simulink model "model_linearization"  (R2014b)
settings: Solver=ode45  StartTime=0.0  StopTime=10.0  RelTol=1e-3
values from neighbouring files (symbols this model uses):
  states_IC = [      13.9 ... (first row only)    [startup.m]    (also in trim_model.m = [14.048)
undefined symbols (not defined in the file or in its folder): slparams
settings Model: Creator=thomas  LastModifiedBy=thomas

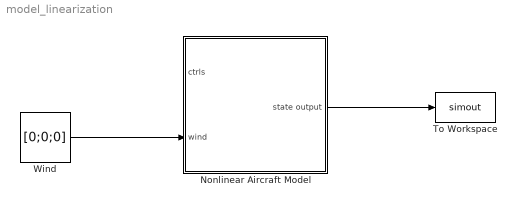
== system model_linearization ==
  Nonlinear Aircraft Model : Subsystem
  To Workspace : ToWorkspace  VariableName=simout  SampleTime=-1
  Wind : Constant  Value=[0;0;0]
  wires:
  Wind/1 -> Nonlinear Aircraft Model/2(wind)
  Nonlinear Aircraft Model/1(state output) -> To Workspace/1

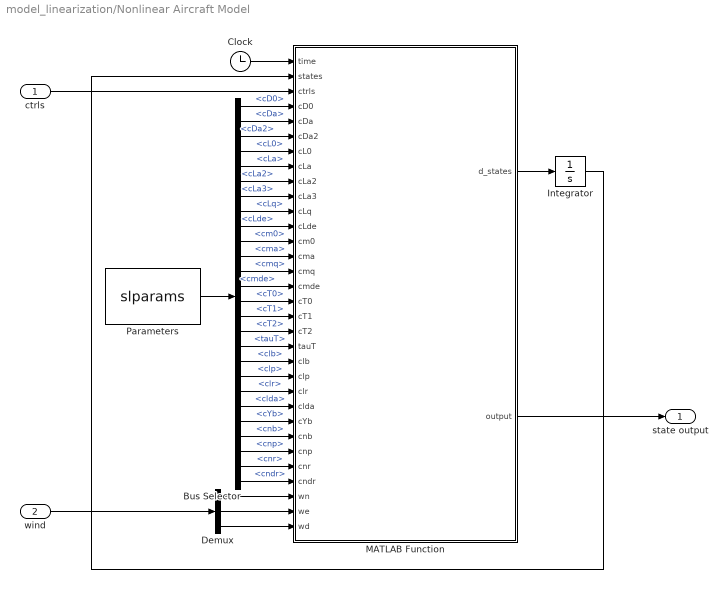
== system model_linearization/Nonlinear Aircraft Model ==
  ctrls : Inport
  wind : Inport  Port=2
  Bus Selector : BusSelector  OutputSignals=cD0,cDa,cDa2,cL0,cLa,cLa2,cLa3,cLq,cLde,cm0,cma,cmq,cmde,cT0,cT1,cT2,tauT,clb,clp,clr,clda,cYb,cnb,cnp,cnr,cndr
  Clock : Clock
  Demux : Demux  Outputs=3
  Integrator : Integrator  InitialCondition=states_IC
  MATLAB Function : MATLAB Function  TreatAsAtomicUnit=on
  Parameters : Constant  Value=slparams  OutDataTypeStr=Bus: slBus1
  state output : Outport
  wires:
  Bus Selector/3 -> MATLAB Function/6(cDa2)  "<cDa2>"
  Bus Selector/8 -> MATLAB Function/11(cLq)  "<cLq>"
  Bus Selector/5 -> MATLAB Function/8(cLa)  "<cLa>"
  Bus Selector/16 -> MATLAB Function/19(cT2)  "<cT2>"
  Bus Selector/13 -> MATLAB Function/16(cmde)  "<cmde>"
  Bus Selector/1 -> MATLAB Function/4(cD0)  "<cD0>"
  Bus Selector/17 -> MATLAB Function/20(tauT)  "<tauT>"
  Bus Selector/2 -> MATLAB Function/5(cDa)  "<cDa>"
  Bus Selector/11 -> MATLAB Function/14(cma)  "<cma>"
  Bus Selector/20 -> MATLAB Function/23(clr)  "<clr>"
  Bus Selector/21 -> MATLAB Function/24(clda)  "<clda>"
  Bus Selector/18 -> MATLAB Function/21(clb)  "<clb>"
  Bus Selector/15 -> MATLAB Function/18(cT1)  "<cT1>"
  Bus Selector/6 -> MATLAB Function/9(cLa2)  "<cLa2>"
  Bus Selector/4 -> MATLAB Function/7(cL0)  "<cL0>"
  Bus Selector/22 -> MATLAB Function/25(cYb)  "<cYb>"
  Bus Selector/26 -> MATLAB Function/29(cndr)  "<cndr>"
  Bus Selector/23 -> MATLAB Function/26(cnb)  "<cnb>"
  Bus Selector/10 -> MATLAB Function/13(cm0)  "<cm0>"
  Bus Selector/25 -> MATLAB Function/28(cnr)  "<cnr>"
  Bus Selector/9 -> MATLAB Function/12(cLde)  "<cLde>"
  Bus Selector/24 -> MATLAB Function/27(cnp)  "<cnp>"
  Bus Selector/19 -> MATLAB Function/22(clp)  "<clp>"
  Parameters/1 -> Bus Selector/1
  Bus Selector/7 -> MATLAB Function/10(cLa3)  "<cLa3>"
  Bus Selector/14 -> MATLAB Function/17(cT0)  "<cT0>"
  Bus Selector/12 -> MATLAB Function/15(cmq)  "<cmq>"
  MATLAB Function/1(d_states) -> Integrator/1
  ctrls/1 -> MATLAB Function/3(ctrls)
  Integrator/1 -> MATLAB Function/2(states)
  MATLAB Function/2(output) -> state output/1
  Clock/1 -> MATLAB Function/1(time)
  wind/1 -> Demux/1
  Demux/1 -> MATLAB Function/30(wn)
  Demux/2 -> MATLAB Function/31(we)
  Demux/3 -> MATLAB Function/32(wd)

== matlab function model_linearization/Nonlinear Aircraft Model/MATLAB Function ==
  data: time input; d_states output; states input; ctrls input; cD0 input; cDa input; cDa2 input; cL0 input; cLa input; cLa2 input; cLa3 input; cLq input; cLde input; cm0 input; cma input; cmq input; cmde input; cT0 input; cT1 input; cT2 input; tauT input; clb input; clp input; clr input; clda input; cYb input; cnb input; cnp input; cnr input; cndr input; wn input; we input; wd input; output output
function [d_states, output]  = NonlinearModel(time, states, ctrls,...
    cD0, cDa, cDa2, ...
    cL0, cLa, cLa2, cLa3, cLq, cLde, ...
    cm0, cma, cmq, cmde, ...
    cT0, cT1, cT2, tauT, ...
    clb, clp, clr, clda, ...
    cYb, ...
    cnb, cnp, cnr, cndr, ...
    wn, we, wd)

%#codegen
%--------------------------------------------------------------------------
% TECHPOD NONLINEAR 6DoF AIRCRAFT MODEL
%
% last update 07.06.15, Thomas Stastny

%--------------------------------------------------------------------------

% states
u       = states(1);    % x-body velocity
v       = states(2);    % y-body velocity
w       = states(3);    % z-body velocity

p       = states(4);    % roll rate
q       = states(5);    % pitch rate
r       = states(6);    % yaw rate

phi 	= states(7);    % roll angle
theta   = states(8);    % pitch angle
psi     = states(9);    % flight path angle

n       = states(10);   % inertial north position
e       = states(11);   % inertial east position
d       = states(12);   % inertial down position

uT      = states(13);

% controls
uTcmd      = ctrls(1);     % throttle
uE      = ctrls(2);     % elevator deflection
uA      = ctrls(3);     % aileron deflection (uniform)
uR      = ctrls(4);     % rudder deflection

if uTcmd>1, uTcmd=1; end;
if uTcmd<0, uTcmd=0; end;
if uE>20*pi/180, uE=20*pi/180; end;
if uE<-20*pi/180, uE=-20*pi/180; end;
if uA>20*pi/180, uA=20*pi/180; end;
if uA<-20*pi/180, uA=-20*pi/180; end;
if uR>20*pi/180, uR=20*pi/180; end;
if uR<-20*pi/180, uR=-20*pi/180; end;

% MODEL CONSTRUCTION ------------------------------------------------------

% intermediate states
V       = sqrt(u^2+v^2+w^2);
beta    = asin(v/V);
alpha   = atan(w/u);

% MODEL CONSTRUCTION ------------------------------------------------------

% geometry
S_wing          = 0.47;     % wing surface              [m^2]
b_wing          = 2.59;     % wingspan                  [m]
c_chord         = 0.180;    % mean chord length         [m]
i_thrust        = 0*pi/180;	% thrust incidence angle    [rad] -->NOTE: i is defined from body x in positive pitch (up)

% mass / inertia
mass    = 2.65;         % total mass of airplane    [kg]
Ixx     = 0.1512*1.1;	% inertias                  [kg m^2]
Iyy     = 0.2785*1.4;	% inertias                  [kg m^2]
Izz     = 0.3745*1.4;	% inertias                  [kg m^2]
Ixz     = 0.0755;       % inertias                  [kg m^2]

% environment
g       = 9.81;     % gravitational acceleration    [m/s^2]
rho_air = 1.18;     % air density

% wind to body transform
ca = cos(alpha);
sa = sin(alpha);
H_W2B = [ca,	0,	-sa;
         0,     1,	0;
         sa,    0,	ca];

% non-dimensionalization
p_hat	= p*b_wing /(2*V);
q_hat	= q*c_chord /(2*V);
r_hat	= r*b_wing /(2*V);
q_bar_S = 1/2*rho_air*V^2*S_wing;

% stability axis aerodynamic force coefficients
cD      = cD0 + cDa*alpha + cDa2*alpha^2;
cY_s    = cYb*beta;
cL      = cL0 + cLa*alpha + cLa2*alpha^2 + cLa3*alpha^3 + cLq*q_hat + cLde*uE;

% body frame aerodynamic forces
cXYZ    = H_W2B*[-cD; cY_s; -cL];
X       = q_bar_S * cXYZ(1);
Y       = q_bar_S * cXYZ(2);
Z       = q_bar_S * cXYZ(3);

% stability axis aerodynamic moment coefficients
cl_s    = clb*beta + clp*p_hat + clr*r_hat + clda*uA;
cm_s    = cm0 + cma*alpha + cmq*q_hat + cmde*uE;
cn_s    = cnb*beta + cnp*p_hat + cnr*r_hat + cndr*uR;

% body frame aerodynamic moments
clmn    = H_W2B*[cl_s; cm_s; cn_s];
Lm      = q_bar_S * b_wing * clmn(1);
Mm      = q_bar_S * c_chord * clmn(2);
Nm      = q_bar_S * b_wing * clmn(3);
     
% thrust force
uT_dot = uTcmd/tauT - uT/tauT;
T   = cT0 + cT1*uT + cT2*uT^2;                                                              % neglecting 2nd order term

% intermediate state differentials
u_dot       = r*v - q*w - g*sin(theta) + (X+T*cos(i_thrust))/mass;
v_dot       = p*w - r*u + g*sin(phi)*cos(theta) + Y/mass;
w_dot       = q*u - p*v + g*cos(phi)*cos(theta) + (Z+T*sin(i_thrust))/mass;

% state differentials
% V_dot       = (u*u_dot + v*v_dot + w*w_dot)/V;
% beta_dot    = (V*v_dot - v*V_dot)/(V^2*cos(beta));
% alpha_dot   = (u*w_dot - w*u_dot)/(u^2 + w^2);

I1          = Ixz*(Iyy-Ixx-Izz);
I2          = (Ixx*Izz-Ixz^2);
p_dot       = (Izz*Lm+Ixz*Nm-(I1*p+(Ixz^2+Izz*(Izz-Iyy))*r)*q)/I2;
q_dot       = (Mm-(Ixx-Izz)*p*r-Ixz*(p^2-r^2))/Iyy;                        % neglecting thrusting moments
r_dot       = (Ixz*Lm+Ixx*Nm+(I1*r+(Ixz^2+Ixx*(Ixx-Iyy))*p)*q)/I2;

phi_dot     = p + (q*sin(phi) + r*cos(phi))*tan(theta);
theta_dot   = q*cos(phi) - r*sin(phi);
psi_dot     = (q*sin(phi) + r*cos(phi))/cos(theta);

n_dot       = u*cos(theta)*cos(psi)+v*(sin(phi)*sin(theta)*cos(psi)-...
    cos(phi)*sin(psi))+w*(sin(phi)*sin(psi)+cos(phi)*sin(theta)*cos(psi)) + wn;
e_dot       = u*cos(theta)*sin(psi)+v*(cos(phi)*cos(psi)+sin(phi)*sin(theta)*sin(psi))+...
    w*(cos(phi)*sin(theta)*sin(psi)-sin(phi)*cos(psi)) + we;
d_dot       = -u*sin(theta)+v*sin(phi)*cos(theta)+w*cos(phi)*cos(theta) + wd;

gamma = -asin(d_dot/sqrt(n_dot^2+e_dot^2+d_dot^2));

% DIFFERENTIAL STATES/OUTPUTS ---------------------------------------------

% d_states
d_states = zeros(13,1);
d_states(1)     = u_dot;
d_states(2)     = v_dot;
d_states(3)     = w_dot;
d_states(4)     = p_dot;
d_states(5)     = q_dot;
d_states(6)     = r_dot;
d_states(7)     = phi_dot;
d_states(8)     = theta_dot;
d_states(9)     = psi_dot;
d_states(10)    = n_dot;
d_states(11)    = e_dot;
d_states(12)    = d_dot;
d_states(13)    = uT_dot;

% output
output = zeros(13,1);
output(1)	= V;
output(2)	= beta;
output(3)	= alpha;
output(4)	= p;
output(5)	= q;
output(6)	= r;
output(7)	= phi;
output(8)	= theta;
output(9)   = psi;
output(10)  = n;
output(11)  = e;
output(12)  = d;
output(13) = uT;
